simulink model "KetQuaMoPhong"  (R2023b)
settings: Solver=FixedStepAuto  StartTime=0  StopTime=2475  FixedStep=0.005  RelTol=1e-3
undefined symbols (not defined in the file): Ion, Lithium
libraries: fl_lib x6, spsMosfetLib x6, nesl_utility x4, sdl_lib x3, spsBatteryLib x1, spsSeriesRLCBranchLib x1, autolibshared x1, spsPermanentMagnetSynchronousMachineLib x1, slpidlib x1, sps_lib x1
settings Model: Creator=Tefilus  LastModifiedBy=Tefilus
settings DataIOCC: ReturnWorkspaceOutputs=off

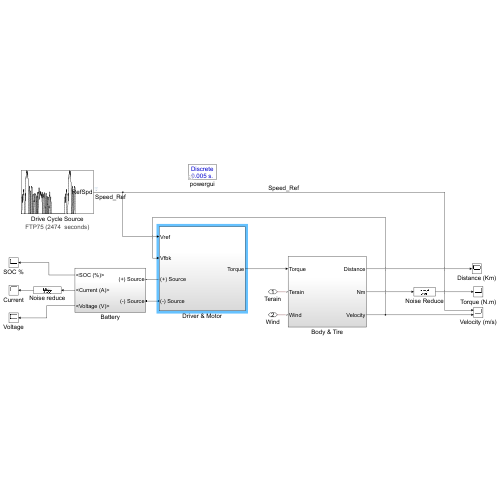
[thumbnail: Simulink's stored preview of the top-level diagram]
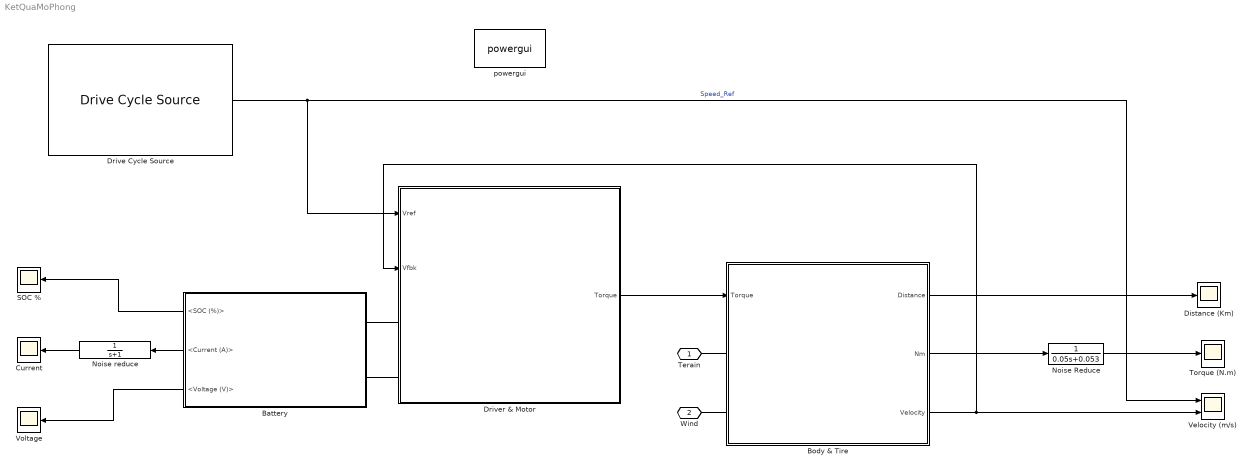
== system KetQuaMoPhong ==
  Battery : Subsystem
  Body & Tire : Subsystem
  Current : Scope
  Distance (Km) : Scope
  Drive Cycle Source : autolibshared/Drive Cycle Source  cycleVar=FTP75  fileVar=NYCC.txt  tfinal="2474  seconds"  cycleRepeat=off  outAccPort=off  outGearPort=off  gearList=No gear data  t_wot1=5  xdot_woto=0  xdot_wot1=30  t_wot2=20  xdot_wot2=0  t_wotend=30  srcUnit=m/s  outUnit=m/s  srcAccUnit=m/s/s  outAccUnit=m/s^2  dt=0  aMode=1  faultOption=off  velBnd=2  velBndUnit=mph  inUnit=m/s  timeBnd=1  failOption=off  stopSim=off  maxFaultCnt=10  maxFaultTime=2  maxTotFaultTime=15  traceOption=off  dtTrace=1  traceWindow=10  lastDCname=FTP75  lastOutUnit=mph  lastDT=0  lastTB=1  lastSB=2  forceCalcBound=off
  Driver & Motor : Subsystem
  Noise Reduce : TransferFcn  Denominator=[0.05 0.053]  ParameterTunability=Optimized
  Noise reduce : TransferFcn  Denominator=[1 1]
  SOC % : Scope
  Torque (N.m) : Scope
  Velocity (m/s) : Scope  NumInputPorts=2
  Voltage : Scope
  powergui : sps_lib/powergui  Priority=1  SimulationMode=Discrete  SampleTime=0.005  frequency=60  Iterations=50  frequencyindice=0  Pbase=100e6  ErrMax=1e-4  UnitsV=kV  UnitsW=MW  buscounter=0  FunctionMessages=off  echomessages=off  EnableUseOfTLC=off  CurrentSourceSwitches=off  DisableSnubberDevices=off  DisableRonSwitches=off  DisableVfSwitches=off  DisplayEquations=off  AutomaticDiscreteSolvers=off  SolverType=Tustin/Backward Euler (TBE)  Interpol=off  ExternalGateDelay=off  methode=off  Ts=100  x0status=blocks  SPID=on  SwTol=0  HookPort=off  NonlinearTolerance=1e-4  nMaxIteration=100  ContinueOnMaxIteration=off  RestoreLinks=warning  ResistiveCurrentMeasurement=off  Frange=[0:2:500]  Ylog=off  Xlog=on  ShowGrid=off  save=off  variable=ZData  structure=0  ZoomFFT=off  StartTime=0.0  cycles=1  DisplayStyle=1  fundamental=60  FreqAxis=off  MaxFrequency=1000  frequencyindicesteady=1  RmsSteady=1  display=off
  Terain : PMIOPort  Side=Left
  Wind : PMIOPort  Port=2  Side=Left
  wires:
  Battery/1(<SOC (%)>) -> SOC %/1
  Battery/3(<Voltage (V)>) -> Voltage/1
  Drive Cycle Source/1 -> Velocity (m/s)/1, Driver & Motor/1(Vref)  "Speed_Ref"
  Battery/2(<Current (A)>) -> Noise reduce/1
  Noise Reduce/1 -> Torque (N.m)/1
  Noise reduce/1 -> Current/1
  Driver & Motor/1(Torque) -> Body & Tire/1(Torque)
  Body & Tire/2(Nm) -> Noise Reduce/1
  Body & Tire/1(Distance) -> Distance (Km)/1
  Body & Tire/3(Velocity) -> Driver & Motor/2(Vfbk), Velocity (m/s)/2
  connections:
  Driver & Motor/LConn1 -- Battery/LConn1
  Driver & Motor/LConn2 -- Battery/LConn2
  Terain/RConn1 -- Body & Tire/LConn1
  Wind/RConn1 -- Body & Tire/LConn2

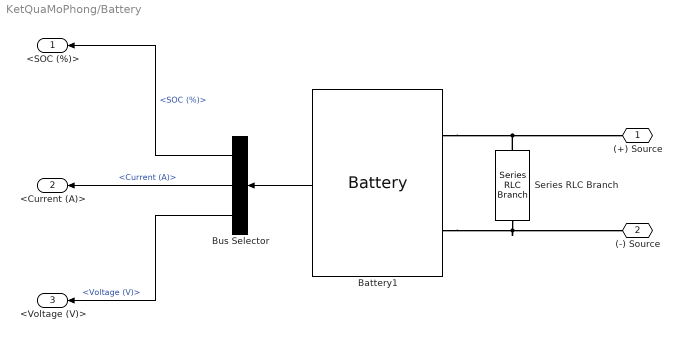
== system KetQuaMoPhong/Battery ==
  Battery1 : spsBatteryLib/Battery  BatType=Lithium-Ion  ShowTempParam=off  ThermalPreset=no  ShowAgeParam=off  NomV=50.4  NomQ=22  SOC=100  Batt_Tr=30  PresetModel=on  MaxQ=22  MinV=37.8  FullV=58.665  Dis_rate=9.5652  R=0.022909  Normal_OP=19.8957  expZone="[54.4514      1.08087]"  current=[6.5 13 32.5]  Units=Time  Tci=20  NomT=20  T2=-30  MaxQ2=4.8  FullV2=7.1  Normal_OP2=5.655  expZone2="[6.58           1]"  Rca=0.6  ti=2000  Dp=0  Neq0=0  Tsim=1e6  Ta1=25  Qeol=5.4*0.9  Reol=0.013333*1.2  Char_age=[2.3478, 3]  Dis_age=[2.3478, 10]  N1=1500  N2=10500  N3=1000  N4=1400  Ta2=45  N5=950
  Bus Selector : BusSelector  OutputSignals=SOC (%),Current (A),Voltage (V)
  Series RLC Branch : spsSeriesRLCBranchLib/Series RLC Branch  LConnTagsString=__new0  RConnTagsString=__new0  BranchType=C  Resistance=1  Inductance=1e-3  SetiL0=off  InitialCurrent=0  Capacitance=75e-3  Setx0=off  InitialVoltage=0  Measurements=None
  (+) Source : PMIOPort  Side=Left
  (-) Source : PMIOPort  Port=2  Side=Left
  <SOC (%)> : Outport
  <Current (A)> : Outport  Port=2
  <Voltage (V)> : Outport  Port=3
  wires:
  Battery1/1 -> Bus Selector/1
  Bus Selector/3 -> <Voltage (V)>/1  "<Voltage (V)>"
  Bus Selector/2 -> <Current (A)>/1  "<Current (A)>"
  Bus Selector/1 -> <SOC (%)>/1  "<SOC (%)>"
  connections:
  Battery1/LConn1 -- Series RLC Branch/LConn1 -- (+) Source/RConn1
  Battery1/LConn2 -- Series RLC Branch/RConn1 -- (-) Source/RConn1

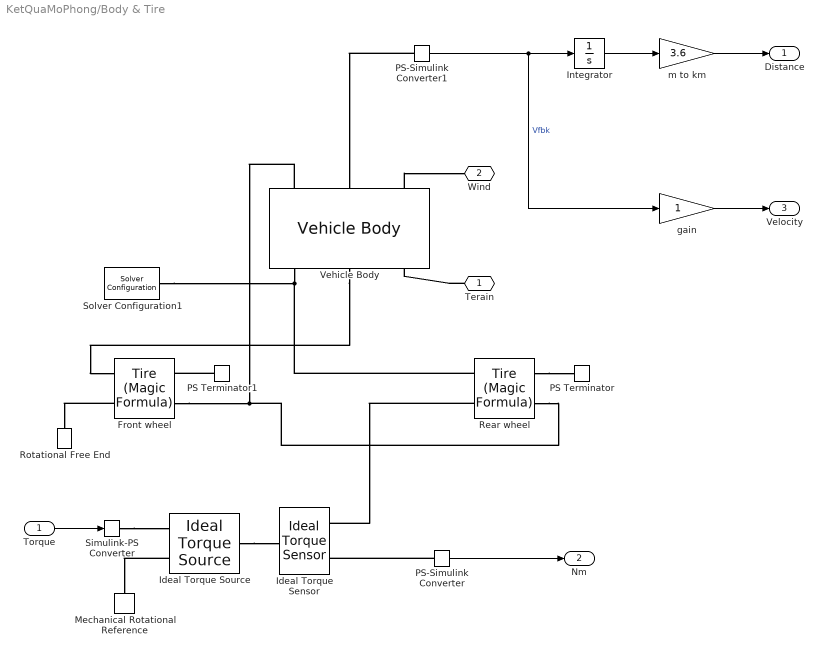
== system KetQuaMoPhong/Body & Tire ==
  Torque : Inport
  Front wheel : sdl_lib/Tires & Vehicles/Tire (Magic Formula)  parameterization=sdl.enum.magic_tire_model.peak  F_z1=3000 N  F_x1=3500 N  kappa1=10  B_m=10  C_m=1.9  D_m=1  E_m=0.97  fz0=4000 N  p_Cx=1.685  p_Dx=[1.21, -.037]  p_Ex=[.344, .095, -.02, 0]  p_Kx=[21.51, -.163, .245]  p_Hx=[-.002, .002]  p_Vx=[0, 0]  rolling_radius_model=sdl.enum.RollingRadiusParameterization.Constant  r_e=0.22 m  r_0=0.3 m  breff=8.39  dreff=0.26  freff=0.074  q_re0=0.99  q_v1=0.008  longvl=17 m/s  cz=5e5 N/m  model_resistance=true  resistance_model=sdl.enum.rollingResistanceParameterization.constant  coeff=0.005  p_tire=250e3 Pa  alpha=-0.003  beta=0.97  coeff_a=84e-4  coeff_b=6.2e-4 s/m  coeff_c=1.6e-4 s^2/m^2  p_tire0=240e3 Pa  fz0_resistance=4000 N  vH0=16 m/s  q_Sy=[.0082, 0, .0014, .001, 0, 0, 1.08, -.5]  v_thr=0.001 m/s  enable_scaling_coefficients=false  lfzO=1  lcx=1  lmux=1  lex=1  lkx=1  lhx=1  lvx=1  lmy=1  model_compliance=sdl.enum.compliance.off  stiffness=1e6 N/m  damping=1000 N*s/m  model_inertia=sdl.enum.model_inertia.off  inertia=1 kg*m^2  initial_velocity=0 rad/s  vxlow=1 m/s  v_tr_thr=0.1*0.1 m/s  kpumin=-1e5  kpumax=1e5
  Ideal Torque Sensor : fl_lib/Mechanical/Mechanical Sensors/Ideal Torque Sensor
  Ideal Torque Source : fl_lib/Mechanical/Mechanical Sources/Ideal Torque Source
  Integrator : Integrator
  Mechanical Rotational Reference : fl_lib/Mechanical/Rotational Elements/Mechanical Rotational Reference
  PS Terminator : fl_lib/Physical Signals/Sinks/PS Terminator
  PS Terminator1 : fl_lib/Physical Signals/Sinks/PS Terminator
  PS-Simulink Converter : nesl_utility/PS-Simulink Converter  PhysicalDomain=network_engine_domain  SubClassName=ps_output  LeftPortType=input  RightPortType=output  PseudoPeriodic=off  Frequencies=[]  VectorFormat=inherit  Unit=inherit  AffineConversion=off
  PS-Simulink Converter1 : nesl_utility/PS-Simulink Converter  PhysicalDomain=network_engine_domain  SubClassName=ps_output  LeftPortType=input  RightPortType=output  PseudoPeriodic=off  Frequencies=[]  VectorFormat=inherit  Unit=inherit  AffineConversion=off
  Rear wheel : sdl_lib/Tires & Vehicles/Tire (Magic Formula)  parameterization=sdl.enum.magic_tire_model.peak  F_z1=3000 N  F_x1=3500 N  kappa1=10  B_m=10  C_m=1.9  D_m=1  E_m=0.97  fz0=4000 N  p_Cx=1.685  p_Dx=[1.21, -.037]  p_Ex=[.344, .095, -.02, 0]  p_Kx=[21.51, -.163, .245]  p_Hx=[-.002, .002]  p_Vx=[0, 0]  rolling_radius_model=sdl.enum.RollingRadiusParameterization.Constant  r_e=0.22 m  r_0=0.3 m  breff=8.39  dreff=0.26  freff=0.074  q_re0=0.99  q_v1=0.008  longvl=17 m/s  cz=5e5 N/m  model_resistance=true  resistance_model=sdl.enum.rollingResistanceParameterization.constant  coeff=0.005  p_tire=250e3 Pa  alpha=-0.003  beta=0.97  coeff_a=84e-4  coeff_b=6.2e-4 s/m  coeff_c=1.6e-4 s^2/m^2  p_tire0=240e3 Pa  fz0_resistance=4000 N  vH0=16 m/s  q_Sy=[.0082, 0, .0014, .001, 0, 0, 1.08, -.5]  v_thr=0.001 m/s  enable_scaling_coefficients=false  lfzO=1  lcx=1  lmux=1  lex=1  lkx=1  lhx=1  lvx=1  lmy=1  model_compliance=sdl.enum.compliance.off  stiffness=1e6 N/m  damping=1000 N*s/m  model_inertia=sdl.enum.model_inertia.off  inertia=1 kg*m^2  initial_velocity=0 rad/s  vxlow=1 m/s  v_tr_thr=0.1*0.1 m/s  kpumin=-1e5  kpumax=1e5
  Rotational Free End : fl_lib/Mechanical/Rotational Elements/Rotational Free End  w_specify=off  w_priority=None  w=0 rad/s  w_nominal_specify=off  w_nominal_unit=rad/s  w_nominal_value=1
  Simulink-PS Converter : nesl_utility/Simulink-PS Converter  PhysicalDomain=network_engine_domain  SubClassName=ps_input  LeftPortType=input  RightPortType=output  PseudoPeriodic=off  Frequencies=[]  NoiseDistribution=none  NoiseParameters=[]  Unit=1  AffineConversion=off  FilteringAndDerivatives=provide  SimscapeFilterOrder=1  InputFilterTimeConstant=0.001  UdotUserProvided=0
  Solver Configuration1 : nesl_utility/Solver Configuration  PhysicalDomain=network_engine_domain  SubClassName=solver  LeftPortType=input  RightPortType=generic  Tones=[]  Harmonics=[]  SimulateNoise=off  Profile=off  UseLocalSampling=off  EnableSwitchedLinearOptims=on  FrequencyDomain=off  UseCCode=off  RelTol=0.001  AbsTol=1e-06  MinStep=1e-09  ToWorkspace=off  RevertToSquareIcSolve=off  NumHomotopyIterations=100  PhasorMode=off  PhasorModeNumHarmonics=1  ConsistencySolver=NEWTON_FTOL  IndexReductionMethod=DerivativeReplacement  DoDC=off  ResidualTolerance=1e-09  ConsistencyTolSource=GLOBAL  ConsistencyAbsTol=0.001  ConsistencyRelTol=0.001  ConsistencyTolFactor=0.001  UseLocalSolver=off  LocalSolverChoice=NE_BACKWARD_EULER_ADVANCER  ResolveIndetEquations=on  FunctionEvalNumThread=1  LocalSolverSampleTime=0.001  DoFixedCost=off  MaxNonlinIter=3  MaxModeIter=2  ComputeImpulses=off  ImpulseIterations=2  LinearAlgebra=auto  LinearAlgebraNumThread=0  EquationFormulation=NE_TIME_EF  DelaysMemoryBudget=1024  AutomaticFiltering=on  FilteringTimeConstant=0.001  PartitionStorageMethod=AS_NEEDED  PartitionMemoryBudget=1024  PartitionMethod=ROBUST  MultibodyUseLocalSolver=off  MultibodyLocalSolverChoice=ODE1  MultibodyLocalSolverSampleTime=0.001
  Vehicle Body : sdl_lib/Tires & Vehicles/Vehicle Body  mass=70 kg  n_w=1  x_f=0.6 m  x_r=0.7 m  y_c=0.155 m  mass_var=simscape.enum.onoff.off  g=9.81 m/s^2  liftoff_warning=simscape.enum.onoff.off  area=0.76 m^2  Cd=0.2  rho=1.18 kg/m^3  model_pitch=simscape.enum.onoff.off  inertia=4000 kg*m^2  suspension_model=sdl.enum.linearTLU.linear  k_f=1e4 N/m  b_f=1e4 N*s/m  k_r=1e4 N/m  b_r=1e4 N*s/m  k_f_TLU=[-2000, -1000, 0, 1000, 2000] N  x_f_TLU=[-.4, -.2, 0, .2, .4] m  b_f_TLU=[-200, -100, 0, 100, 200] N  v_f_TLU=[-4, -2, 0, 2, 4] m/s  k_r_TLU=[-2000, -1000, 0, 1000, 2000] N  x_r_TLU=[-.4, -.2, 0, .2, .4] m  b_r_TLU=[-200, -100, 0, 100, 200] N  v_r_TLU=[-4, -2, 0, 2, 4] m/s  interp_method=simscape.enum.interpolation.linear  extrap_method=simscape.enum.extrapolation.linear  model_hardstop=simscape.enum.onoff.off  upper_bound_f=.25 m  lower_bound_f=-.25 m  stop_k_f=1e6 N/m  stop_b_f=150 N*s/m  upper_bound_r=.25 m  lower_bound_r=-.25 m  stop_k_r=1e6 N/m  stop_b_r=150 N*s/m  initial_pitch=0 rad  initial_pitch_rate=0 rad/s  v_specify=on  v_priority=High  v=0 m/s  v_nominal_specify=off  v_nominal_unit=m/s  v_nominal_value=1
  "gain " : Gain
  m to km : Gain  Gain=3.6
  Terain : PMIOPort  Side=Left
  Wind : PMIOPort  Port=2  Side=Left
  Distance : Outport
  Nm : Outport  Port=2
  Velocity : Outport  Port=3
  wires:
  PS-Simulink Converter1/1 -> "gain "/1, Integrator/1  "Vfbk"
  Integrator/1 -> m to km/1
  PS-Simulink Converter/1 -> Nm/1
  Torque/1 -> Simulink-PS Converter/1
  m to km/1 -> Distance/1
  "gain "/1 -> Velocity/1
  connections:
  PS-Simulink Converter1/LConn1 -- Vehicle Body/LConn2
  Front wheel/LConn2 -- Rotational Free End/LConn1
  PS-Simulink Converter/LConn1 -- Ideal Torque Sensor/RConn2
  Front wheel/RConn2 -- Rear wheel/RConn2 -- Vehicle Body/LConn1
  Vehicle Body/RConn1 -- Solver Configuration1/RConn1 -- Rear wheel/LConn1
  Ideal Torque Source/RConn2 -- Mechanical Rotational Reference/LConn1
  Ideal Torque Source/LConn1 -- Ideal Torque Sensor/LConn1
  Simulink-PS Converter/RConn1 -- Ideal Torque Source/RConn1
  Rear wheel/RConn1 -- PS Terminator/LConn1
  Vehicle Body/LConn3 -- Wind/RConn1
  Vehicle Body/RConn2 -- Front wheel/LConn1
  PS Terminator1/LConn1 -- Front wheel/RConn1
  Rear wheel/LConn2 -- Ideal Torque Sensor/RConn1
  Terain/RConn1 -- Vehicle Body/RConn3

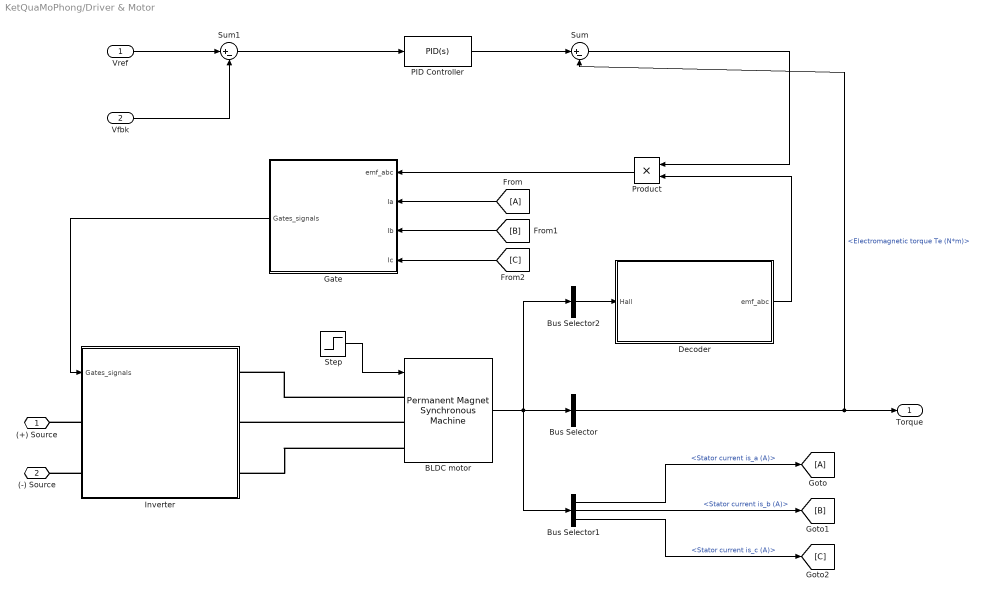
== system KetQuaMoPhong/Driver & Motor ==
  Vref : Inport
  Vfbk : Inport  Port=2
  BLDC motor : spsPermanentMagnetSynchronousMachineLib/Permanent Magnet Synchronous Machine  NbPhases=3  FluxDistribution=Sinusoidal  RotorType=Round  MechanicalLoad=Speed w  PresetModel=No  ShowDetailedParameters=on  MeasurementBus=off  Resistance=0.18  Inductance=8.5e-3  dqInductances=[8.5e-3, 8.5e-3]  La=0.000835  MachineConstant=Flux linkage established by magnets (V.s)  Flux=0.0714394  VoltageCst=51.8307  TorqueCst=0.42864  Flat=120  Mechanical=[0.000621417 0.000303448 4]  PolePairs=4  InitialConditions=[0,0, 0,0]  InitialConditions5ph=[0 0 0 0 0 0]  RefAngle=90 degrees behind phase A axis (modified Park)  IterativeDiscreteModel=Trapezoidal robust  TsBlock=-1  TsPowergui=0
  Bus Selector : BusSelector  OutputSignals=Electromagnetic torque Te (N*m)
  Bus Selector1 : BusSelector  OutputSignals=Stator current is_a (A),Stator current is_b (A),Stator current is_c (A)
  Bus Selector2 : BusSelector  OutputSignals=Hall effect signal h_a,Hall effect signal h_b,Hall effect signal h_c  OutputAsBus=on
  Decoder : Subsystem
  From : From
  Gate : Subsystem
  Goto : Goto
  Inverter : Subsystem
  PID Controller : slpidlib/PID Controller  Controller=PID  Form=Parallel  TimeDomain=Continuous-time  UseExternalTs=off  SampleTime=-1  IntegratorMethod=Forward Euler  FilterMethod=Forward Euler  ControllerParametersSource=internal  P=100  I=0.001  UseKiTs=off  D=0.05  N=100  UseFilter=on  TunerSelectOption=Transfer Function Based (PID Tuner App)  InitialConditionSource=internal  InitialConditionForIntegrator=0  InitialConditionForFilter=0  DifferentiatorICPrevScaledInput=0  ExternalReset=none  IgnoreLimit=on  TrackingMode=off  Kt=1  LimitOutput=on  SatLimitsSource=internal  UpperSaturationLimit=1000  LowerSaturationLimit=-200  LinearizeAsGain=on  AntiWindupMode=none  Kb=1  LimitIntegrator=off  UpperIntegratorSaturationLimit=inf  LowerIntegratorSaturationLimit=-inf  POutMin=[]  POutMax=[]  IOutMin=[]  IOutMax=[]  DOutMin=[]  DOutMax=[]  NOutMin=[]  NOutMax=[]  SumOutMin=[]  SumOutMax=[]  SaturationOutMin=[]  SaturationOutMax=[]  PParamMin=[]  PParamMax=[]  IParamMin=[]  IParamMax=[]  DParamMin=[]  DParamMax=[]  NParamMin=[]  NParamMax=[]  KbParamMin=[]  KbParamMax=[]  KtParamMin=[]  KtParamMax=[]  KbOutMin=[]  KbOutMax=[]  KtOutMin=[]  KtOutMax=[]  IntegratorOutMin=[]  IntegratorOutMax=[]  FilterOutMin=[]  FilterOutMax=[]  SumI1OutMin=[]  SumI1OutMax=[]  SumI2OutMin=[]  SumI2OutMax=[]  SumI3OutMin=[]  SumI3OutMax=[]  SumI4OutMin=[]  SumI4OutMax=[]  SumDOutMin=[]  SumDOutMax=[]  DifferentiatorOutMin=[]  DifferentiatorOutMax=[]  FilterDiffOutCoefMin=[]  FilterDiffOutCoefMax=[]  ReciprocalOutMin=[]  ReciprocalOutMax=[]  SumDenOutMin=[]  SumDenOutMax=[]  SumNumOutMin=[]  SumNumOutMax=[]  DivideOutMin=[]  DivideOutMax=[]  UdiffTsProdOutMin=[]  UdiffTsProdOutMax=[]  NTsProdOutMin=[]  NTsProdOutMax=[]  UintegralTsProdOutMin=[]  UintegralTsProdOutMax=[]  UngainTsProdOutMin=[]  UngainTsProdOutMax=[]  ClampingZeroOutDataTypeStr=Inherit: Inherit via back propagation  ClampingZeroOutMin=[]  ClampingZeroOutMax=[]  FilterDenConstantOutDataTypeStr=Inherit: Inherit via back propagation  FilterDenConstantOutMin=[]  FilterDenConstantOutMax=[]  PCopyOutDataTypeStr=Inherit: Inherit via back propagation  PCopyOutMin=[]  PCopyOutMax=[]  NCopyOutDataTypeStr=Inherit: Inherit via back propagation  NCopyOutMin=[]  NCopyOutMax=[]  IntegratorContinuousStateAttributes=''  IntegratorStateMustResolveToSignalObject=off  IntegratorRTWStateStorageClass=Auto  FilterContinuousStateAttributes=''  FilterStateMustResolveToSignalObject=off  FilterRTWStateStorageClass=Auto  ParallelPVariant=InternalParameters  IdealPVariant=Disabled  IVariant=InternalParameters  DVariant=InternalParameters  IntegratorVariant=Continuous  SatVariant=Enabled  AWVariant=Passthrough  PCopyVariant=Disabled  TRVariant=Disabled  FdbkBlocksVariant=Forward  IdealPFdbkVariant=Disabled  SatFdbkVariant=Disabled  DerivativeFilterVariant=ContFilter  NVariant=InternalParameters  NCopyVariant=Disabled  FilterICVariant=InternalICsFilter  IntegratorICVariant=InternalICs  ExternalResetVariant=Disabled  TRSumVariant=Passthrough  SumFdbkVariant=Disabled  SumVariant=Sum_PID  TsampFilterVariant=InternalTs  TsampNgainVariant=Passthrough  TsampIntegralVariant=Disabled_SignalSpec  ExternalSaturationOutDataTypeStr=Inherit: Same as second input
  Product : Product
  Step : Step  Time=0  After=10  SampleTime=0
  Sum : Sum  Inputs=|+-
  Sum1 : Sum  Inputs=|+-
  (+) Source : PMIOPort  Side=Left
  (-) Source : PMIOPort  Port=2  Side=Left
  Torque : Outport
  wires:
  Sum1/1 -> PID Controller/1
  Step/1 -> BLDC motor/1
  From/1 -> Gate/2(Ia)
  Bus Selector1/3 -> [C]  "<Stator current is_c (A)>"
  [C] -> Gate/4(Ic)
  Vfbk/1 -> Sum1/2
  PID Controller/1 -> Sum/1
  Bus Selector/1 -> Torque/1, Sum/2  "<Electromagnetic torque Te (N*m)>"
  Sum/1 -> Product/1
  Bus Selector1/2 -> [B]  "<Stator current is_b (A)>"
  [B] -> Gate/3(Ib)
  Gate/1(Gates_signals) -> Inverter/1(Gates_signals)
  Bus Selector1/1 -> Goto/1  "<Stator current is_a (A)>"
  BLDC motor/1 -> Bus Selector/1, Bus Selector1/1, Bus Selector2/1
  Vref/1 -> Sum1/1
  Decoder/1(emf_abc) -> Product/2
  Bus Selector2/1 -> Decoder/1(Hall)
  Product/1 -> Gate/1(emf_abc)
  connections:
  BLDC motor/LConn2 -- Inverter/RConn2
  BLDC motor/LConn1 -- Inverter/RConn1
  Inverter/LConn2 -- (-) Source/RConn1
  Inverter/LConn1 -- (+) Source/RConn1
  BLDC motor/LConn3 -- Inverter/RConn3

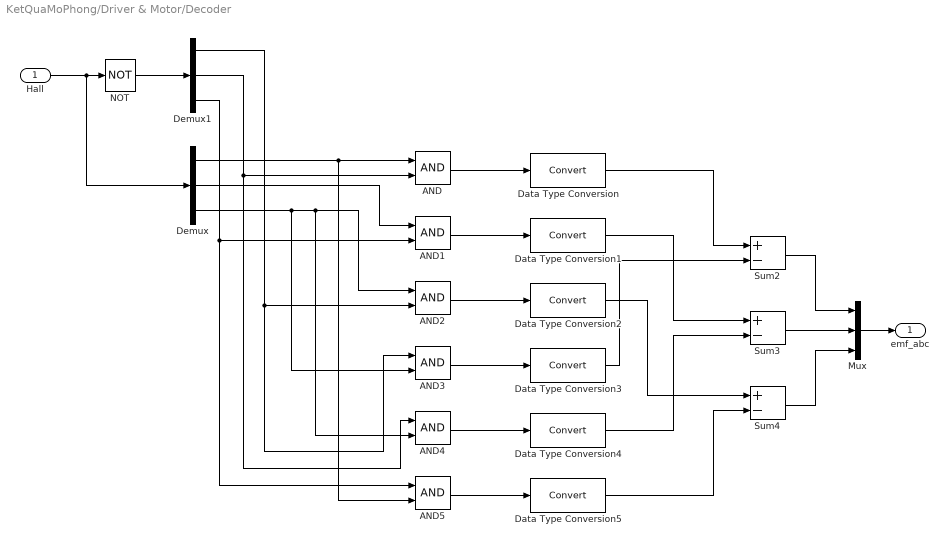
== system KetQuaMoPhong/Driver & Motor/Decoder ==
  Hall : Inport
  AND{,1..5} (6 alike) : Logic  AllPortsSameDT=off  OutDataTypeStr=boolean
  Data Type Conversion{,1..5} (6 alike) : DataTypeConversion  SaturateOnIntegerOverflow=off  RndMeth=Floor
  Demux : Demux  Outputs=3
  Demux1 : Demux  Outputs=3
  Mux : Mux  Inputs=3
  NOT : Logic  Operator=NOT  AllPortsSameDT=off  OutDataTypeStr=boolean
  Sum2 : Sum  Inputs=+-
  Sum3 : Sum  Inputs=+-
  Sum4 : Sum  Inputs=+-
  emf_abc : Outport
  wires:
  Sum3/1 -> Mux/2
  AND3/1 -> Data Type Conversion3/1
  NOT/1 -> Demux1/1
  Demux1/3 -> AND5/1, AND1/2
  Data Type Conversion5/1 -> Sum4/2
  Data Type Conversion3/1 -> Sum2/2
  Demux1/1 -> AND2/2, AND3/1
  Demux/1 -> AND/1, AND5/2
  Demux/3 -> AND3/2, AND2/1, AND4/2
  Demux1/2 -> AND/2, AND4/1
  AND2/1 -> Data Type Conversion2/1
  Sum4/1 -> Mux/3
  AND1/1 -> Data Type Conversion1/1
  Mux/1 -> emf_abc/1
  Hall/1 -> Demux/1, NOT/1
  AND4/1 -> Data Type Conversion4/1
  Data Type Conversion1/1 -> Sum3/1
  AND/1 -> Data Type Conversion/1
  Sum2/1 -> Mux/1
  Data Type Conversion4/1 -> Sum3/2
  AND5/1 -> Data Type Conversion5/1
  Data Type Conversion2/1 -> Sum4/1
  Demux/2 -> AND1/1
  Data Type Conversion/1 -> Sum2/1

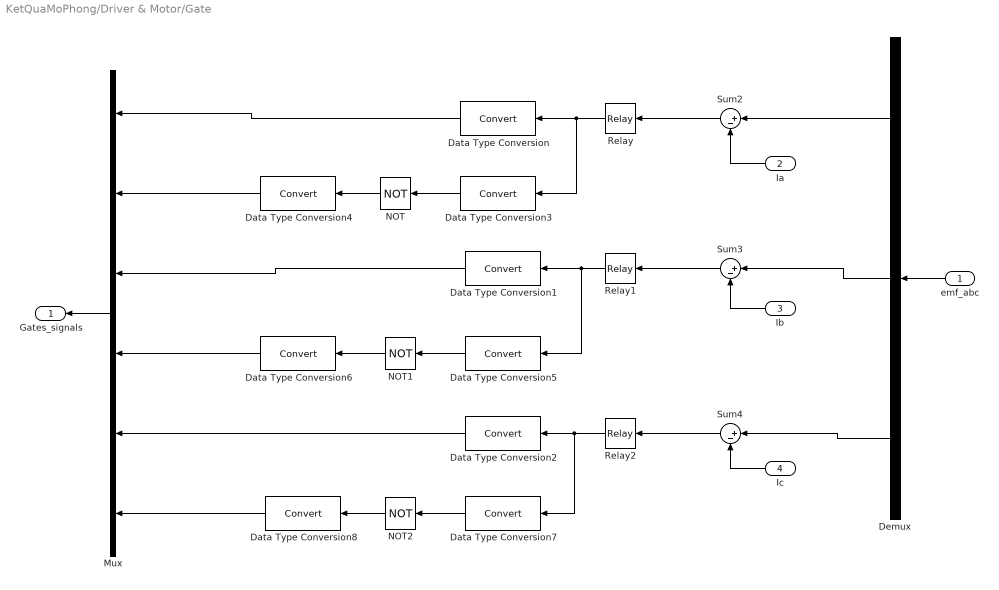
== system KetQuaMoPhong/Driver & Motor/Gate ==
  emf_abc : Inport
  Ia : Inport  Port=2
  Ib : Inport  Port=3
  Ic : Inport  Port=4
  Data Type Conversion{,1..8} (9 alike) : DataTypeConversion
  Demux : Demux  Outputs=3
  Mux : Mux  Inputs=6
  NOT : Logic  Operator=NOT  AllPortsSameDT=off  OutDataTypeStr=boolean
  NOT1 : Logic  Operator=NOT  AllPortsSameDT=off  OutDataTypeStr=boolean
  NOT2 : Logic  Operator=NOT  AllPortsSameDT=off  OutDataTypeStr=boolean
  Relay : Relay  OnSwitchValue=0.1  OffSwitchValue=-0.1
  Relay1 : Relay  OnSwitchValue=0.1  OffSwitchValue=-0.1
  Relay2 : Relay  OnSwitchValue=0.1  OffSwitchValue=-0.1
  Sum2 : Sum  Inputs=|+-
  Sum3 : Sum  Inputs=|+-
  Sum4 : Sum  Inputs=|+-
  Gates_signals : Outport
  wires:
  Sum3/1 -> Relay1/1
  Relay1/1 -> Data Type Conversion5/1, Data Type Conversion1/1
  Sum4/1 -> Relay2/1
  Relay/1 -> Data Type Conversion3/1, Data Type Conversion/1
  Demux/3 -> Sum4/1
  Demux/1 -> Sum2/1
  Demux/2 -> Sum3/1
  Sum2/1 -> Relay/1
  emf_abc/1 -> Demux/1
  Relay2/1 -> Data Type Conversion7/1, Data Type Conversion2/1
  Ia/1 -> Sum2/2
  Ib/1 -> Sum3/2
  Ic/1 -> Sum4/2
  Data Type Conversion3/1 -> NOT/1
  NOT/1 -> Data Type Conversion4/1
  Data Type Conversion5/1 -> NOT1/1
  NOT1/1 -> Data Type Conversion6/1
  Data Type Conversion7/1 -> NOT2/1
  NOT2/1 -> Data Type Conversion8/1
  Data Type Conversion/1 -> Mux/1
  Data Type Conversion8/1 -> Mux/6
  Data Type Conversion2/1 -> Mux/5
  Data Type Conversion6/1 -> Mux/4
  Data Type Conversion1/1 -> Mux/3
  Data Type Conversion4/1 -> Mux/2
  Mux/1 -> Gates_signals/1

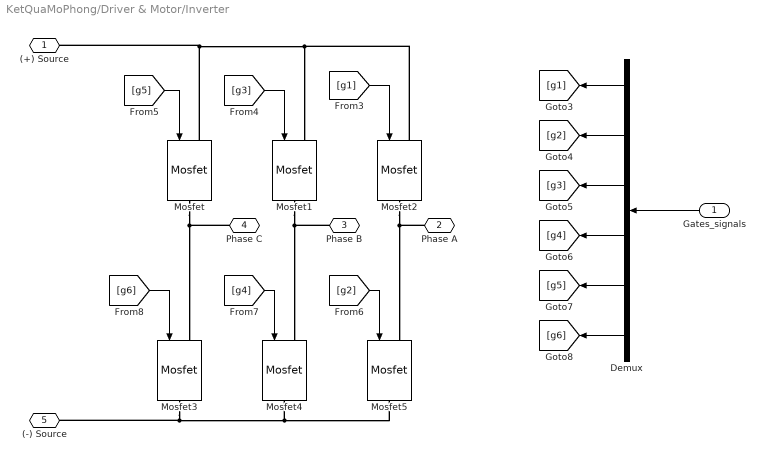
== system KetQuaMoPhong/Driver & Motor/Inverter ==
  Gates_signals : Inport
  Demux : Demux  Outputs=6
  Mosfet{,1..5} (6 alike) : spsMosfetLib/Mosfet  Ron=0.1  Lon=0  Rd=0.01  Vfd=0  IC=0  Rs=1e5  Cs=inf  Measurements=off
  (+) Source : PMIOPort  Side=Left
  Phase A : PMIOPort  Port=2  Side=Right
  Phase B : PMIOPort  Port=3  Side=Right
  Phase C : PMIOPort  Port=4  Side=Right
  (-) Source : PMIOPort  Port=5  Side=Left
  wires:
  Demux/1 -> [g1]
  Demux/4 -> [g4]
  Demux/6 -> [g6]
  Demux/5 -> [g5]
  [g6] -> Mosfet3/1
  [g4] -> Mosfet4/1
  Demux/3 -> [g3]
  Demux/2 -> [g2]
  [g1] -> Mosfet2/1
  [g3] -> Mosfet1/1
  [g5] -> Mosfet/1
  Gates_signals/1 -> Demux/1
  [g2] -> Mosfet5/1
  connections:
  Mosfet1/RConn1 -- Phase B/RConn1 -- Mosfet4/LConn1
  Mosfet/LConn1 -- (+) Source/RConn1 -- Mosfet2/LConn1 -- Mosfet1/LConn1
  Mosfet/RConn1 -- Phase C/RConn1 -- Mosfet3/LConn1
  Mosfet2/RConn1 -- Phase A/RConn1 -- Mosfet5/LConn1
  Mosfet3/RConn1 -- (-) Source/RConn1 -- Mosfet4/RConn1 -- Mosfet5/RConn1
